simulink model "a71really"  (R2016a)
settings: Solver=VariableStepAuto  StartTime=0.0  StopTime=10.0  RelTol=1e-3
values from neighbouring files (symbols this model uses):
  D = ones(3)    [a2.m]    (also in a71test.m = 0)
  I = zeros(10,10)    [a2.m]    (also in a71test.m = 60)
  M_L1 = 0    [a71test.m]
  M_L2 = 6.01    [a71test.m]
  n_soll = 20.1    [a71test.m]
  P = 0    [a71test.m]
  t_ML_step = 12    [DCTEST.m]    (also in a71test.m = 3)
  t_n_soll_step = 0.5    [a71test.m]
libraries: a71real x1, simulink x1
settings Model: Creator=mam1205  LastModifiedBy=mam1205

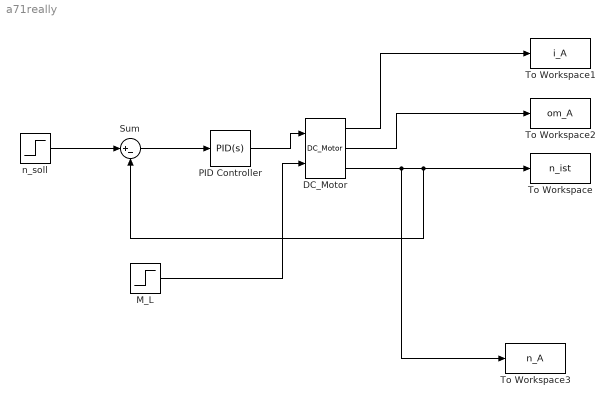
== system a71really ==
  "DC_Motor " : a71real/DC_Motor 
  M_L : Step  Time=t_ML_step  Before=M_L1  After=M_L2  SampleTime=0
      settings: AttributesFormatString=|
      | %<Before>
      | %<After>
      | %<Time>
  PID Controller : simulink/Continuous/PID Controller  Controller=PID  TimeDomain=Continuous-time  SampleTime=-1  IntegratorMethod=Forward Euler  FilterMethod=Forward Euler  Form=Parallel  UseFilter=on  ControllerParametersSource=internal  P=P  I=I  D=D  N=100  InitialConditionSource=internal  InitialConditionForIntegrator=0  InitialConditionForFilter=0  ExternalReset=none  LimitOutput=off  UpperSaturationLimit=inf  LowerSaturationLimit=-inf  LinearizeAsGain=on  AntiWindupMode=none  Kb=1  TrackingMode=off  Kt=1  PParamMin=[]  PParamMax=[]  IParamMin=[]  IParamMax=[]  DParamMin=[]  DParamMax=[]  NParamMin=[]  NParamMax=[]  KbParamMin=[]  KbParamMax=[]  KtParamMin=[]  KtParamMax=[]  POutMin=[]  POutMax=[]  IOutMin=[]  IOutMax=[]  DOutMin=[]  DOutMax=[]  NOutMin=[]  NOutMax=[]  KbOutMin=[]  KbOutMax=[]  KtOutMin=[]  KtOutMax=[]  IntegratorOutMin=[]  IntegratorOutMax=[]  FilterOutMin=[]  FilterOutMax=[]  SumOutMin=[]  SumOutMax=[]  SumI1OutMin=[]  SumI1OutMax=[]  SumI2OutMin=[]  SumI2OutMax=[]  SumI3OutMin=[]  SumI3OutMax=[]  SumDOutMin=[]  SumDOutMax=[]  SaturationOutMin=[]  SaturationOutMax=[]  IntegratorContinuousStateAttributes=''  IntegratorStateMustResolveToSignalObject=off  IntegratorRTWStateStorageClass=Auto  FilterContinuousStateAttributes=''  FilterStateMustResolveToSignalObject=off  FilterRTWStateStorageClass=Auto  DifferentiatorICPrevScaledInput=0  DifferentiatorOutMin=[]  DifferentiatorOutMax=[]
  Sum : Sum  Inputs=|+-
  To Workspace : ToWorkspace  VariableName=n_ist  SaveFormat=Timeseries  SampleTime=-1
  To Workspace1 : ToWorkspace  VariableName=i_A  SaveFormat=Timeseries  SampleTime=-1
  To Workspace2 : ToWorkspace  VariableName=om_A  SaveFormat=Timeseries  SampleTime=-1
  To Workspace3 : ToWorkspace  VariableName=n_A  SaveFormat=Timeseries  SampleTime=-1
  n_soll : Step  Time=t_n_soll_step  After=n_soll  SampleTime=0
      settings: AttributesFormatString=|
      | %<Before>
      | %<After>
      | %<Time>
  wires:
  n_soll/1 -> Sum/1
  Sum/1 -> PID Controller/1
  "DC_Motor "/3 -> To Workspace/1, Sum/2, To Workspace3/1
  "DC_Motor "/1 -> To Workspace1/1
  "DC_Motor "/2 -> To Workspace2/1
  PID Controller/1 -> "DC_Motor "/1
  M_L/1 -> "DC_Motor "/2
